simulink model "dstatcom"  (Simulink 7.9)
settings: Solver=FixedStepDiscrete  SolverMode=SingleTasking  StartTime=0.0  StopTime=0.5  FixedStep=Ts  RelTol=1e-3
InitFcn:
  |  Ts=5e-6;
undefined symbols (not defined in the file): D11, Delta, DiscIntNeverNeededParam
libraries: powerlib x39, powerlib_extras x25
(part 2 of 2)

== system dstatcom/DStatcom/Controller/PWM Modulator /SubSystem ==
  note: (or B or C)
  note: (or B or C)
  note: |
      | |
      | |
      | |
      | |
      | |
      | |
      | |
      | |
      | |
      | |
      | |
      | |
      | |
      | |
      | |
      | |
      | |
      | |
      | |
      | |
      | |
      | |
      | |
      | |
      | |
      | |
      | |
  note: Pulse pattern identical to Bridge 1
  note: Bridge 2
  note: Pulses P2 -->
  note: Pulse pattern identical to Bridge 1
  note: Bridge 2
  note: Pulses P2 -->
  note: 12: Q4 (phase C)
  note: 11: Q3 (phase C)
  note: 10: Q2 (phase C)
  note: 9: Q1 (phase C )
  note: 8: Q4 (phase B)
  note: 7: Q3 (phase B)
  note: 6: Q2 (phase B)
  note: 5: Q1 (phase B )
  note: Bridge 1
  note: 4: Q4 (phase A)
  note: 3: Q3 (phase A)
  note: 2: Q2 (phase A)
  note: 1: Q1 (phase A )
  note: Pulses P1 -->
  note: 6: Q2 (phase C)
  note: Bridge 1
  note: 5: Q1 (phase C)
  note: 4: Q2 (phase B)
  note: 3: Q1 (phase B)
  note: 2: Q2 (phase A)
  note: 1: Q1 (phase A )
  note: Pulses P1 -->
  note: 3-level
  note: 2-level
  note: 0 -------------------------
  note: |
      | |
      | |
      | |
      | |
      | [Q2]
      | |
      | |
      | |
      | |
  note: |
      | |
      | |
      | |
      | |
      | [Q1]
      | |
      | |
      | |
      | |
  note: Vdc --------------------
  note: ------------ A
  note: + Vdc --------------------------
  note: - Vdc--------------------------
  note: N -----------
  note: |
      | |
      | |
      | |
      | |
      | |
      | |
      | |
      | |
      | |
      | |
  note: ---------- A
  note: ----------[D]---------
  note: ----------[D]---------
  note: |
      | |
      | [Q4]
      | |
      | |
      | |
  note: |
      | |
      | [Q3]
      | |
      | |
  note: |
      | |
      | [Q2]
      | |
      | |
  note: |
      | |
      | |
      | [Q1]
      | |
      | |

== system dstatcom/DStatcom/Controller/PWM Modulator /2-level Type/Carriers Generator ==
  theta : Inport  PortDimensions=3
  Gain1 : Gain  Gain=2/pi  SaturateOnIntegerOverflow=on  OutDataTypeStr=Inherit: Same as input  ParamDataTypeStr=Inherit: Same as input
  Trigonometric Function : Trigonometry  Operator=asin
  Trigonometric Function3 : Trigonometry
  C : Outport
  wires:
  Gain1/1 -> C/1  "Carrier"
  theta/1 -> Trigonometric Function3/1
  Trigonometric Function3/1 -> Trigonometric Function/1
  Trigonometric Function/1 -> Gain1/1

== system dstatcom/DStatcom/Controller/PWM Modulator /3-level Type/Carriers Generator ==
  theta : Inport  PortDimensions=3
  Constant2 : Constant  Value=0.5
  Gain1 : Gain  Gain=1/pi  SaturateOnIntegerOverflow=on  OutDataTypeStr=Inherit: Same as input  ParamDataTypeStr=Inherit: Same as input
  Sum1 : Sum  SaturateOnIntegerOverflow=on  InputSameDT=on  OutDataTypeStr=Inherit: Same as first input
  Sum2 : Sum  Inputs=+-  SaturateOnIntegerOverflow=on  InputSameDT=on  OutDataTypeStr=Inherit: Same as first input
  Trigonometric Function : Trigonometry  Operator=asin
  Trigonometric Function3 : Trigonometry
  C+ : Outport
  C- : Outport  Port=2
  wires:
  Trigonometric Function/1 -> Gain1/1
  Trigonometric Function3/1 -> Trigonometric Function/1
  Gain1/1 -> Sum1/1, Sum2/1
  Constant2/1 -> Sum2/2, Sum1/2
  Sum2/1 -> C-/1  "Carrier 1-"
  Sum1/1 -> C+/1  "Carrier 1+"
  theta/1 -> Trigonometric Function3/1

== system dstatcom/DStatcom/Controller/PWM Modulator /3-level Type/State-to-Pulses Decoder ==
  note: + Vdc --------------------------
  note: - Vdc--------------------------
  note: N -----------
  note: |
      | |
      | |
      | |
      | |
      | |
      | |
      | |
      | |
      | |
      | |
  note: ---------- A
  note: ----------[D]---------
  note: ----------[D]---------
  note: |
      | |
      | [Q4]
      | |
      | |
      | |
  note: |
      | |
      | [Q3]
      | |
      | |
  note: |
      | |
      | [Q2]
      | |
      | |
  note: |
      | |
      | |
      | [Q1]
      | |
      | |
  note: Phase C: 9 to 12
  note: Phase A: 1 to 4
  note: Phase B: 5 to 8
  note: 3-phase State-to-Pulses Decoder
  note: --------------------------------------------------------------
  note: |
      | |
      | |
      | |
      | |
      | |
      | |
      | |
      | |
  note: 1
  note: 1
  note: 0
  note: 0
  note: -1
  note: 0
  note: 1
  note: 1
  note: 0
  note: 0
  note: Q4
  note: Q3
  note: Q2
  note: Q1
  note: 0
  note: 0
  note: 1
  note: 1
  note: Firing pulses
  note: 1
  note: State
  State : Inport  PortDimensions=3
  Constant11 : Constant  Value=[1 1 0 0]
  Constant12 : Constant  Value=[0 0 1 1]
  Constant13 : Constant  Value=[0 1 1 0]
  Constant2 : Constant  Value=2
  Demux : Demux  Outputs=3
  Multiport Switch : MultiPortSwitch  zeroidx=off  SaturateOnIntegerOverflow=on  InputSameDT=on
  Multiport Switch3 : MultiPortSwitch  zeroidx=off  SaturateOnIntegerOverflow=on  InputSameDT=on
  Multiport Switch4 : MultiPortSwitch  zeroidx=off  SaturateOnIntegerOverflow=on  InputSameDT=on
  Mux : Mux  Inputs=[4 4 4]
  Sum : Sum  SaturateOnIntegerOverflow=on  InputSameDT=on  OutDataTypeStr=Inherit: Same as first input
  Pulses : Outport
  wires:
  Multiport Switch4/1 -> Mux/3
  Multiport Switch3/1 -> Mux/2
  Multiport Switch/1 -> Mux/1
  Constant11/1 -> Multiport Switch4/4, Multiport Switch3/4, Multiport Switch/4
  Constant13/1 -> Multiport Switch4/3, Multiport Switch3/3, Multiport Switch/3
  Constant12/1 -> Multiport Switch4/2, Multiport Switch3/2, Multiport Switch/2
  Demux/3 -> Multiport Switch4/1
  Demux/2 -> Multiport Switch3/1
  Demux/1 -> Multiport Switch/1
  Constant2/1 -> Sum/2
  State/1 -> Sum/1
  Sum/1 -> Demux/1
  Mux/1 -> Pulses/1

== system dstatcom/DStatcom/Controller/PWM Modulator /3-level Type/State-to-Pulses Decoder1 ==
  note: State
  note: 1
  note: Firing pulses
  note: 1
  note: 1
  note: 0
  note: 0
  note: Q1
  note: Q2
  note: Q3
  note: Q4
  note: 0
  note: 0
  note: 1
  note: 1
  note: 0
  note: -1
  note: 0
  note: 0
  note: 1
  note: 1
  note: |
      | |
      | |
      | |
      | |
      | |
      | |
      | |
      | |
  note: --------------------------------------------------------------
  note: 3-phase State-to-Pulses Decoder
  note: Phase B: 5 to 8
  note: Phase A: 1 to 4
  note: Phase C: 9 to 12
  note: |
      | |
      | |
      | [Q1]
      | |
      | |
  note: |
      | |
      | [Q2]
      | |
      | |
  note: |
      | |
      | [Q3]
      | |
      | |
  note: |
      | |
      | [Q4]
      | |
      | |
      | |
  note: ----------[D]---------
  note: ----------[D]---------
  note: ---------- A
  note: |
      | |
      | |
      | |
      | |
      | |
      | |
      | |
      | |
      | |
      | |
  note: N -----------
  note: - Vdc--------------------------
  note: + Vdc --------------------------
  State : Inport  PortDimensions=3
  Constant11 : Constant  Value=[1 1 0 0]
  Constant12 : Constant  Value=[0 0 1 1]
  Constant13 : Constant  Value=[0 1 1 0]
  Constant2 : Constant  Value=2
  Demux : Demux  Outputs=3
  Multiport Switch : MultiPortSwitch  zeroidx=off  SaturateOnIntegerOverflow=on  InputSameDT=on
  Multiport Switch3 : MultiPortSwitch  zeroidx=off  SaturateOnIntegerOverflow=on  InputSameDT=on
  Multiport Switch4 : MultiPortSwitch  zeroidx=off  SaturateOnIntegerOverflow=on  InputSameDT=on
  Mux : Mux  Inputs=[4 4 4]
  Sum : Sum  SaturateOnIntegerOverflow=on  InputSameDT=on  OutDataTypeStr=Inherit: Same as first input
  Pulses : Outport
  wires:
  Mux/1 -> Pulses/1
  Sum/1 -> Demux/1
  State/1 -> Sum/1
  Constant2/1 -> Sum/2
  Demux/1 -> Multiport Switch/1
  Demux/2 -> Multiport Switch3/1
  Demux/3 -> Multiport Switch4/1
  Constant12/1 -> Multiport Switch/2, Multiport Switch3/2, Multiport Switch4/2
  Constant13/1 -> Multiport Switch/3, Multiport Switch3/3, Multiport Switch4/3
  Constant11/1 -> Multiport Switch/4, Multiport Switch3/4, Multiport Switch4/4
  Multiport Switch/1 -> Mux/1
  Multiport Switch3/1 -> Mux/2
  Multiport Switch4/1 -> Mux/3
